simulink model "bubblechase"  (R2015a)
settings: Solver=ode4  SolverMode=MultiTasking  StartTime=0.0  StopTime=inf  FixedStep=BKIN_STEP_TIME  RelTol=1e-3
StartFcn:
  |  warndlg('Dexterit-E models cannot run under simulation. Please compile your model and run it from within Dexterit-E.');set_param(bdroot,'SimulationCommand','stop')
model workspace (MAT data in the model file):
  BKIN_STEP_TIME = 0.00025
  col_x = 1
  col_y = 2
  E_TARGET_ON = 3
  LOGICAL_RADIUS = 4
  START_TARGET_COL = 1
  END_TARGET_COL = 2
  DELAY_POSTTRIAL_COL = 6
  E_STAY_CENTER = 2
  VISUAL_RADIUS = 3
  COLOR = 5
  K_SCORETEXT_ROW = 1
  LABEL_HEIGHT = 9
  E_HIT_TARGET = 5
  E_MISS_TARGET = 9
  K_REWARD_VAL = 2
  K_VIS_RAD = 3
  E_REWARD = 6
  WAIT_AT_START_COL = 3
  LABEL = 8
  K_SCORE_TIME = 4
  HAND_VIS_COL = 9
  DO_REWARD_COL = 10
  E_SHOW_SCORE = 17
  DISPLAY_TRIAL_COL = 11
  BKIN_KINEMATIC_FRAME_SIZE = 400
  E_NO_EVENT = 0
  PAUSE_TIME_COL = 4
  MAXREACH_TIME_COL = 5
  TARGET_XVEL_COL = 7
  TARGET_YVEL_COL = 8
  K_POP_TIME = 5
  K_POP_R_EXPAND = 6
  K_POP_FADE = 7
  STROKE_WIDTH = 6
  STROKE_COLOR = 7
  K_MAX_DIST = 8
  E_TARGET_ESCAPE = 11
  E_END_BREAK = 20
  BTN_BREAK = 2
undefined symbols (not defined in the file or in its folder): slselsubs
libraries: Video x4, General x3, slrtlib x3, simulink x2, KINARM_general x1, xpcnilib x1
(part 2 of 2)

== matlab function bubblechase/KINARM_HandInTarget/Embedded MATLAB InsideTarget ==
  settings: fimath=|
      | fimath(...
      | 'RoundMode', 'floor',...
      | 'OverflowMode', 'wrap',...
      | 'ProductMode', 'KeepLSB', 'ProductWordLength', 32,...
      | 'SumMode', 'KeepLSB', 'SumWordLength', 32,...
      | 'CastBeforeSum', false)
  data: handpos input size=2; target_type input; attribcol input; num_targets input; intarget output; Target_Table input; mTgtRow input; mTgtPos input
function intarget = FIsInsideTarget(handpos, target_type, attribcol, num_targets, Target_Table,mTgtRow,mTgtPos)
% all dimensions in m, rad
% arguments:
% handpos: x,y positions of center of target
% attribcol: columns in target table specifying target attributes.
% Specific to Target_Type
%	circle:
%	[X0,Y0,r...,rn] where:
%	X0,Y0 : centre of circle
%	r : logical radius of circle (i.e. radius used to determine 'in' or 'out' of target)
%	rn: logical radius of other targets (e.g. 2nd, 3rd) also specified in target row.
%   Up to 4 targets can be specified in a row
% ellipse:
%	[X0,Y0,a,b,t...,an, bn, tn] where:
%	X0,Y0 : centre of ellipse
%	a,b : major, minor radii of ellipse
%	t : rotation of ellipse in degrees
%	an,bn : major, minor radii of ellipse of other targets (e.g. 2nd, 3rd) also specified in target row
%	tn : rotation of ellipse in degrees of other targets (e.g. 2nd, 3rd) also specified in target row
%   Up to 4 targets can be specified in a row


target_col_x=1;
target_col_y=2;

x=handpos(1);
y=handpos(2);

intarget = zeros(size(Target_Table,1),5);

X0 = Target_Table(:,target_col_x)*0.01;			%Target Table sizes in cm in v1.4
Y0 = Target_Table(:,target_col_y)*0.01;			%Target Table sizes in cm in v1.4

%update the target position for the moving target
if (mTgtRow > 0)
    X0(mTgtRow) = mTgtPos(:,1);
    Y0(mTgtRow) = mTgtPos(:,2);
end

deltax=x-X0;
deltay=y-Y0;

if target_type==1			%circle
    for target=1:num_targets
        r = Target_Table(:,attribcol(target))*0.01;			%Target Table sizes in cm in v1.4
        % simple euclidean distance
        distance2 = deltax.^2 + deltay.^2;					%distance2 is the square of the distance
        intarget(:,target) = (distance2 <= r.^2);
    end
elseif target_type==2		%ellipse
    for target=1:num_targets
        a = Target_Table(:,attribcol(target*3-2))*0.01;			%Target Table sizes in cm in v1.4
        b = Target_Table(:,attribcol(target*3-1))*0.01;			%Target Table sizes in cm in v1.4
        t = Target_Table(:,attribcol(target*3))*(pi / 180.0);	%Target Table angles in degrees in v1.4
        sint=sin(t);
        cost=cos(t);
        xrotate=deltax.*cost+deltay.*sint;		%location of x point in ellipse's coordinate frame
        yrotate=-deltax.*sint+deltay.*cost;		%location of y point in ellipse's coordinate frame
        m=yrotate./xrotate;						%slope of line between the (x,y) to (x0,y0) in ellipse's coordinate frame
        y2sq=1./(1./(m.*a).^2+1./b.^2);			%y2sq is y2^2, where y2 is the intersection of the ellipse and the (x,y) to (x0,y0) line
        intarget(:,target) = (yrotate.^2 <= y2sq);
    end
elseif target_type==3       %rectangle
    for target=1:num_targets
        w = Target_Table(:,attribcol(target*3-2))*0.01;  %width (sizes in cm in v1.4)
        h = Target_Table(:,attribcol(target*3-1))*0.01;  %height (sizes in cm in v1.4)
        
        if attribcol(target*3) > 0
            t = Target_Table(:,attribcol(target*3))*(pi / 180.0);  %angle (angles in degrees in v1.4)
        else
            t = zeros(size(Target_Table, 1), 1);
        end
        
        sint=sin(t);
        cost=cos(t);
        
        xrotate=deltax.*cost + deltay.*sint;   %location of x point in rectangle's coordinate frame
        yrotate=-deltax.*sint + deltay.*cost;  %location of y point in rectangle's coordinate frame
        
        intarget(:,target) = abs(xrotate) <= w/2 & abs(yrotate) <= h/2;
    end
elseif target_type==4       %line
    for target=1:num_targets
        % treat the line like a rectangle of height h and width w
        % determine height (stroke width) in the same fashion as in Show_Target
        if attribcol(target*3-2) == 0                     %0 column index means stroke width of 0
            h = zeros(size(Target_Table, 1), 1);
        elseif attribcol(target*3-2) < 0                  %-ve column index means stroke width of 1mm
            h = ones(size(Target_Table, 1), 1) .* 0.001;
        else
            h = Target_Table(:,attribcol(target*3-2)) * 0.01;  %target table contains width in cm
        end
        
        ex = Target_Table(:,attribcol(target*3-1))*0.01;  %endpoint in x relative to start point (cm)
        ey = Target_Table(:,attribcol(target*3))*0.01;    %endpoint in y relative to start point (cm)
        
        w = sqrt(ex.^2 + ey.^2);                          %width (cm)
        
        % determine the vector from the line's midpoint to the hand position
        handx = deltax - ex/2;
        handy = deltay - ey/2;
        
        t = atan2(ey, ex);                                %calculate angle of the line (rads)
        sint = sin(t);
        cost = cos(t);
        
        xrotate = handx.*cost + handy.*sint;   %location of x point in rectangle's coordinate frame
        yrotate = -handx.*sint + handy.*cost;  %location of y point in rectangle's coordinate frame
        
        intarget(:,target) = abs(xrotate) <= w/2 & abs(yrotate) <= h/2;
    end
elseif target_type==5  % triangle
    for target=1:num_targets
        w = Target_Table(:,attribcol(target*4-3))*0.01;         %length (sizes in cm in v1.4)
        
        % If a height column of 0 is specified, make the triangle equilateral. Otherwise, use the
        % values for height and peak offset from the target table.
        if attribcol(target*4-2) > 0
            h = Target_Table(:,attribcol(target*4-2))*0.01;  %height (sizes in cm in v1.4)
            p = Target_Table(:,attribcol(target*4-1))*0.01;  %peak offset (sizes in cm in v1.4)
        else
            h = w.*sin(pi/3.0);
            p = zeros(size(Target_Table, 1), 1);
        end
        
        if attribcol(target*4) > 0
            t = Target_Table(:,attribcol(target*4))*(pi / 180.0);  %angle (angles in degrees in v1.4)
        else
            t = zeros(size(Target_Table, 1), 1);
        end
        
        sint = sin(t);
        cost = cos(t);
        
        xrotate = deltax.*cost + deltay.*sint;   %location of x point in triangle's coordinate frame
        yrotate = -deltax.*sint + deltay.*cost;  %location of y point in triangle's coordinate frame
        
        % Perform a point-in-triangle test using Barycentric coordinates.
        A = [-w/2 - p/3, -h/3];
        B = [2*p/3, 2*h/3];
        C = [w/2 - p/3, -h/3];
        
        v0 = C - A;
        v1 = B - A;
        v2 = [xrotate, yrotate] - A;
        
        dot00 = v0(:,1) .* v0(:,1) + v0(:,2) .* v0(:,2);
        dot01 = v0(:,1) .* v1(:,1) + v0(:,2) .* v1(:,2);
        dot02 = v0(:,1) .* v2(:,1) + v0(:,2) .* v2(:,2);
        dot11 = v1(:,1) .* v1(:,1) + v1(:,2) .* v1(:,2);
        dot12 = v1(:,1) .* v2(:,1) + v1(:,2) .* v2(:,2);
        
        invDenom = 1 ./ (dot00 .* dot11 - dot01 .* dot01);
        u = (dot11 .* dot02 - dot01 .* dot12) .* invDenom;
        v = (dot00 .* dot12 - dot01 .* dot02) .* invDenom;
        
        intarget(:,target) = (u > 0) & (v > 0) & (u + v < 1);
    end
end

== matlab function bubblechase/MovingTarget/Embedded MATLAB Function ==
  settings: fimath=|
      | fimath(...
      | 'RoundMode', 'floor',...
      | 'OverflowMode', 'wrap',...
      | 'ProductMode', 'KeepLSB', 'ProductWordLength', 32,...
      | 'SumMode', 'KeepLSB', 'SumWordLength', 32,...
      | 'CastBeforeSum', false)
  data: VCODES_IN input; CursorPos output; tgt_state input; tgt_vel input; VCODES output; expand input; fade input
function [CursorPos,VCODES]  = Rotation(VCODES_IN,tgt_state,tgt_vel,expand,fade) %Trial_Protocol, Target_Table,
% This block supports an embeddable subset of the MATLAB language.
% See the help menu for details. 

%This block modifies a target VCODE to imbue it with motion and explosion

% VCODEs are length VCODE_LENGTH.
% All dimensions are units of (m).
% VCODE index definition: 1-5 as the same for all target types
% 1 - Target type
%		1=circle
%		2=ellipse
%       3=rectangle
%		4=line
%       5=triangle
%		6 and higher - not implemented yet
% 2 - status
%		0=off
%	   >0=on
% 3 - x position (m)
% 4 - y position (m)
%
%  9: opacity
%
% For circles:
%  10: radius (m)
%
% For ellipses:
%  10: major radius (m)
%  11: minor radius (m)
%  12: orientation of major axis (rad)
%
% For rectangles:
%  10: length (m)
%  11: height (m)
%  12: orientation (rad) (relative to x, y already shown)
%
% For lines:
%  10: endpoint x-axis coordinate relative to start point (m)
%  11: endpoint y-axis coordinate relative to start point (m)
%
% For triangles:
%  10: length (m)
%  11: height (m)
%  12: offset of peak from midpoint of length (m)
%  13: orientation (rad)
VCODES = VCODES_IN;

if tgt_state > 0  %move the target
    
    VCODES(:,3) = VCODES(:,3) + tgt_vel(1); %if the target is visible, add the x step to the target
    VCODES(:,4) = VCODES(:,4) + tgt_vel(2); %if the target is visible, add the y step to the target
    
end

if tgt_state == 2  %if requested, explode the target by increasing its size
    for a = 1:size(VCODES,1)
        if VCODES(a,1) == 1 %circle
            VCODES(a,10) = VCODES(a,10)*expand;
            
        elseif VCODES(a,1) == 2 %ellipse
            VCODES(a,10) = VCODES(a,10)*expand;
            VCODES(a,11) = VCODES(a,11)*expand;
            
        elseif VCODES(a,1) == 3 %rectangle
            VCODES(a,10) = VCODES(a,10)*expand;
            VCODES(a,11) = VCODES(a,11)*expand;
        %elseif VCODES(a,1) == 4 %line  - we can't explode this kind of target!
        elseif VCODES(a,1) == 5 %triangle
            VCODES(a,10) = VCODES(a,10)*expand;
            VCODES(a,11) = VCODES(a,11)*expand;
        end
    end
    
    VCODES(a,9) = fade;  %opacity is out of 100%
    
end

CursorPos = VCODES(:,3:4);


end

== matlab function bubblechase/KINARM_DistanceFromTarget/Embedded MATLAB WhichHand ==
  settings: fimath=|
      | fimath(...
      | 'RoundMode', 'floor',...
      | 'OverflowMode', 'wrap',...
      | 'ProductMode', 'KeepLSB', 'ProductWordLength', 32,...
      | 'SumMode', 'KeepLSB', 'SumWordLength', 32,...
      | 'CastBeforeSum', false)
  data: use_dominant_hand input; dominant_hand input; hand output
function hand = WhichHand(use_dominant_hand, dominant_hand)

if use_dominant_hand==1				%use the dominant hand
	hand=dominant_hand;		
else
	hand=3-dominant_hand;			%use the non-dominant hand. i.e. if dominant_hand=2, hand=1 and vice-versa
end

== matlab function bubblechase/KINARM_DistanceFromTarget/Embedded MATLAB InsideTarget ==
  settings: fimath=|
      | fimath(...
      | 'RoundMode', 'floor',...
      | 'OverflowMode', 'wrap',...
      | 'ProductMode', 'KeepLSB', 'ProductWordLength', 32,...
      | 'SumMode', 'KeepLSB', 'SumWordLength', 32,...
      | 'CastBeforeSum', false)
  data: handpos input size=2; distance output; Target_Table input; mTgtRow input; mTgtPos input
function distance = Distance(handpos, Target_Table, mTgtRow, mTgtPos)
% all dimensions in m, rad
% arguments:
% handpos: x,y positions of center of target

target_col_x=1;
target_col_y=2;
x=handpos(1);
y=handpos(2);

X0 = Target_Table(:,target_col_x)*0.01;			%Target Table sizes in cm in v1.4
Y0 = Target_Table(:,target_col_y)*0.01;			%Target Table sizes in cm in v1.4

%update the target position for the moving target
if (mTgtRow > 0)
    X0(mTgtRow) = mTgtPos(:,1);
    Y0(mTgtRow) = mTgtPos(:,2);
end

distance = sqrt( (X0 - x).^2 + (Y0 - y).^2 );

== matlab function bubblechase/DisplayText/MATLAB Function ==
  data: VCODE input; score input; VCODE_mod output; fdbk_text input; start_tgt_VCODE input
function VCODE_mod = fcn(VCODE,score,fdbk_text,start_tgt_VCODE)


VCODE_mod = VCODE;

if (fdbk_text == 1)  %if this is 1, default = show the score
       
    
    %score is in cents. potentially need to convert to dollars
    
    if (score < 10)
        text1 = 'You earned ';
        text2 = ' cents!';
        
        textout = [text1 int2char(int32(score)) text2];
        
    elseif (score < 100) %score < $1
        text1 = 'You earned ';
        text2 = ' cents!';
        
        n1 = int32(floor(double(score)/10));  %we need to cast score to a double otherwise the arithmetic is wrong!
        n2 = score - n1*10;
        
        textout = [text1 int2char(int32(n1)) int2char(int32(n2)) text2];
        
    else %score > $1, convert to dollars to keep the score readable
        text1 = 'You earned $';
        text2 = '.';
        text3 = '!';
        
        dollars = int32(floor(double(score)/100));
        if (dollars >= 10) %double digit dollar value
            n1d = int32(floor(double(dollars)/10));
            n2d = dollars - n1d*10;
            textdollars = [int2char(int32(n1d)) int2char(int32(n2d))];
        else %single digit
            textdollars = int2char(int32(dollars));
        end
        
        cents = score-dollars*100;
        if (cents < 10)
            textcents = ['0' int2char(int32(cents))];
        else
            n1 = int32(floor(double(cents)/10));
            n2 = round(cents - n1*10);
            textcents = [int2char(int32(n1)) int2char(int32(n2))];
        end
        
        textout = [text1 textdollars text2 textcents text3];
        
    end
    
elseif (fdbk_text == 2) 
    %print "too fast"
    textout = 'Too Fast!';
    
    
elseif (fdbk_text == -2) 
    %print "too slow"
    
    textout = 'Too Slow!';
elseif (fdbk_text == -1)
    textout = 'You Missed!';
elseif (fdbk_text == 5)
    textout = 'Take a break!';
else
    textout = '';
    
end
    

%the first character is VCODE(15)
%need to translate text into ascii:
textnum = double(textout); %this quickly casts each char into a number

%make sure we won't overflow the VCODE: no more than 50 chars! we will
%clip off anything that overflows.
VCODE_mod(1,15:min([15+length(textout),64])) = textnum(1:min([length(textnum),50])); %write out as many the characters as possible into the VCODE
VCODE_mod(1,min([15+length(textout)+1,64])) = 0;  %terminate the string!

VCODE_mod(1,3) = start_tgt_VCODE(1,3);



function s = int2char(n)

n = mod(n,10); %make sure we only have 1 digit or we will get a weird character!

s = char(n+int32('0')); %// add the character

== matlab function bubblechase/Play Sound/Play sound ==
  data: tone input; output output; beep input; errorbeep input; pop input
function output = fcn(tone,beep,errorbeep,pop)
%#codegen

persistent t last_tone_state
if isempty(t), t = 0; end
if isempty(last_tone_state), last_tone_state = 0; end

trigger = last_tone_state ~= tone;
if trigger > 0
    last_tone_state = tone;
end

output = 0;		% default
if t == 0 && trigger > 0
	% start the playing of the sound.
	t = t + 1;
end

if tone == 1
    data = pop;
elseif tone == 2
    data = beep;
elseif tone == 3
    data = errorbeep;
else 
    t = 0;
    data = 0;
end

if t > 0
	output = data(t);
	if t == length(data)
		t = 0;
	else
		t = t + 1;
	end
end

== matlab function bubblechase/KINARM_DistanceBetweenTargets/Embedded MATLAB InsideTarget ==
  settings: fimath=|
      | fimath(...
      | 'RoundMode', 'floor',...
      | 'OverflowMode', 'wrap',...
      | 'ProductMode', 'KeepLSB', 'ProductWordLength', 32,...
      | 'SumMode', 'KeepLSB', 'SumWordLength', 32,...
      | 'CastBeforeSum', false)
  data: distance output; Target_Table input; mTgtRow input; mTgtPos input
function distance = Distance(Target_Table, mTgtRow, mTgtPos)
% all dimensions in m, rad
% arguments:
% handpos: x,y positions of center of target

target_col_x=1;
target_col_y=2;

X0 = Target_Table(:,target_col_x)*0.01;			%Target Table sizes in cm in v1.4
Y0 = Target_Table(:,target_col_y)*0.01;			%Target Table sizes in cm in v1.4

%update the target position for the moving target
if (mTgtRow > 0)
    X0(mTgtRow) = mTgtPos(:,1);
    Y0(mTgtRow) = mTgtPos(:,2);
end

Xdif = repmat(X0,1,length(X0))-repmat(X0',length(X0),1);
Ydif = repmat(Y0,1,length(Y0))-repmat(Y0',length(Y0),1);

distance = sqrt(Xdif.^2 + Ydif.^2);

== matlab function bubblechase/KINARM_HandInTarget/Embedded MATLAB WhichHand ==
  settings: fimath=|
      | fimath(...
      | 'RoundMode', 'floor',...
      | 'OverflowMode', 'wrap',...
      | 'ProductMode', 'KeepLSB', 'ProductWordLength', 32,...
      | 'SumMode', 'KeepLSB', 'SumWordLength', 32,...
      | 'CastBeforeSum', false)
  data: use_dominant_hand input; dominant_hand input; hand output
function hand = WhichHand(use_dominant_hand, dominant_hand)

if use_dominant_hand==1				%use the dominant hand
	hand=dominant_hand;		
else
	hand=3-dominant_hand;			%use the non-dominant hand. i.e. if dominant_hand=2, hand=1 and vice-versa
end
